simulink model "MATMPC_SIMULINK_SPACEROBOT"  (R2019b)
settings: Solver=ode1  StartTime=0.0  StopTime=10  FixedStep=settings.Ts  RelTol=1e-3
undefined symbols (not defined in the file): indata, opt, settings, x0
libraries: dspindex x3
(part 1 of 2)
settings Model: Creator=chen  LastModifiedBy=ichelikh
settings DataIOCC: ReturnWorkspaceOutputs=off
settings DebuggingCC: ArithmeticOperatorsInVariantConditions=warning
settings SFSimCC: SimUseLocalCustomCode=off  CustomCodeUndefinedFunction=UseInterfaceOnly
settings RTWCC: RTWUseLocalCustomCode=off  CheckMdlBeforeBuild=Error

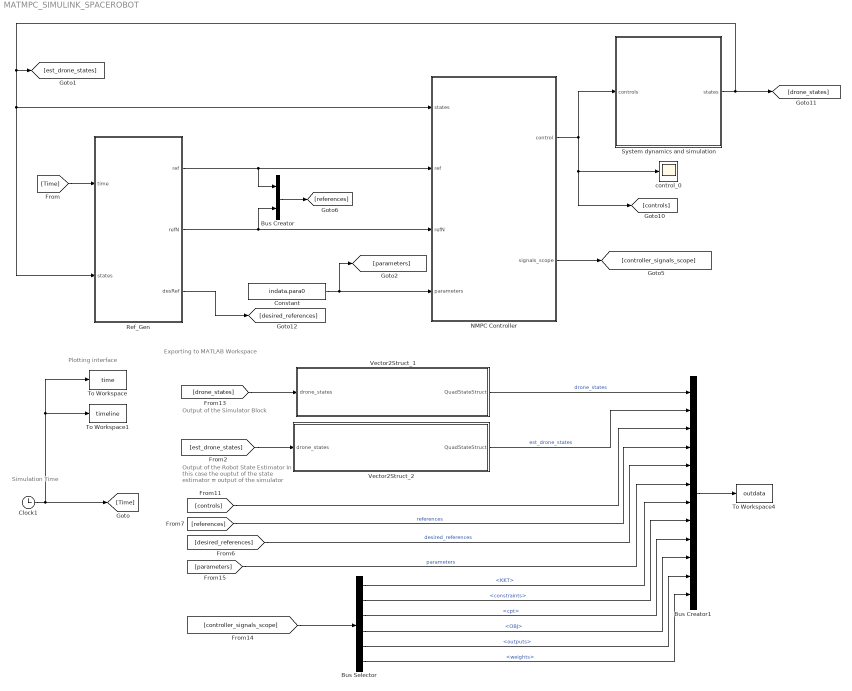
== system MATMPC_SIMULINK_SPACEROBOT ==
  note: Output of the Robot State Estimator
      | In this case the ouptut of the
      | state estimator = output of
      | the simulator
  note: Output of the Simulator Block
  note: Exporting to MATLAB Workspace
  note: Simulation Time
  note: Plotting interface
  Bus Creator : BusCreator  Inputs=2
  Bus Creator1 : BusCreator  Inputs=12
  Bus Selector : BusSelector  OutputSignals=KKT,constraints,cpt,OBJ,outputs,weights
  Clock1 : Clock
  Constant : Constant  Value=indata.para0
  NMPC Controller : Subsystem
  Ref_Gen : Subsystem
  System dynamics and simulation : Subsystem
  To Workspace : ToWorkspace  VariableName=time  SampleTime=-1
      settings: MaxDataPoints=1
  To Workspace1 : ToWorkspace  VariableName=timeline  SampleTime=-1
  To Workspace4 : ToWorkspace  VariableName=outdata  SaveFormat=Timeseries  SampleTime=-1
  Vector2Struct_1 : Subsystem
  Vector2Struct_2 : Subsystem
  control_0 : Scope
  wires:
  NMPC Controller/1(control) -> [controls], control_0/1, System dynamics and simulation/1("controls ")
  Ref_Gen/1(ref) -> Bus Creator/1, NMPC Controller/2("ref ")
  Ref_Gen/2(refN) -> Bus Creator/2, NMPC Controller/3("refN ")
  Constant/1 -> [parameters], NMPC Controller/4(parameters)
  [Time] -> Ref_Gen/1(time)
  Vector2Struct_2/1(QuadStateStruct) -> Bus Creator1/2  "est_drone_states"
  Bus Selector/6 -> Bus Creator1/12  "<weights>"
  Bus Selector/4 -> Bus Creator1/10  "<OBJ>"
  Bus Selector/3 -> Bus Creator1/9  "<cpt>"
  [desired_references] -> Bus Creator1/5  "desired_references"
  [parameters] -> Bus Creator1/6  "parameters"
  [references] -> Bus Creator1/4  "references"
  [controls] -> Bus Creator1/3
  [est_drone_states] -> Vector2Struct_2/1(drone_states)
  Bus Creator1/1 -> To Workspace4/1
  Bus Selector/1 -> Bus Creator1/7  "<KKT>"
  Bus Selector/5 -> Bus Creator1/11  "<outputs>"
  Vector2Struct_1/1(QuadStateStruct) -> Bus Creator1/1  "drone_states"
  Bus Selector/2 -> Bus Creator1/8  "<constraints>"
  [controller_signals_scope] -> Bus Selector/1
  [drone_states] -> Vector2Struct_1/1(drone_states)
  Ref_Gen/3("desRef ") -> [desired_references]
  NMPC Controller/2(signals_scope) -> [controller_signals_scope]
  Bus Creator/1 -> [references]
  System dynamics and simulation/1(states) -> [drone_states], Ref_Gen/2("states "), NMPC Controller/1("states "), [est_drone_states]
  Clock1/1 -> [Time], To Workspace/1, To Workspace1/1

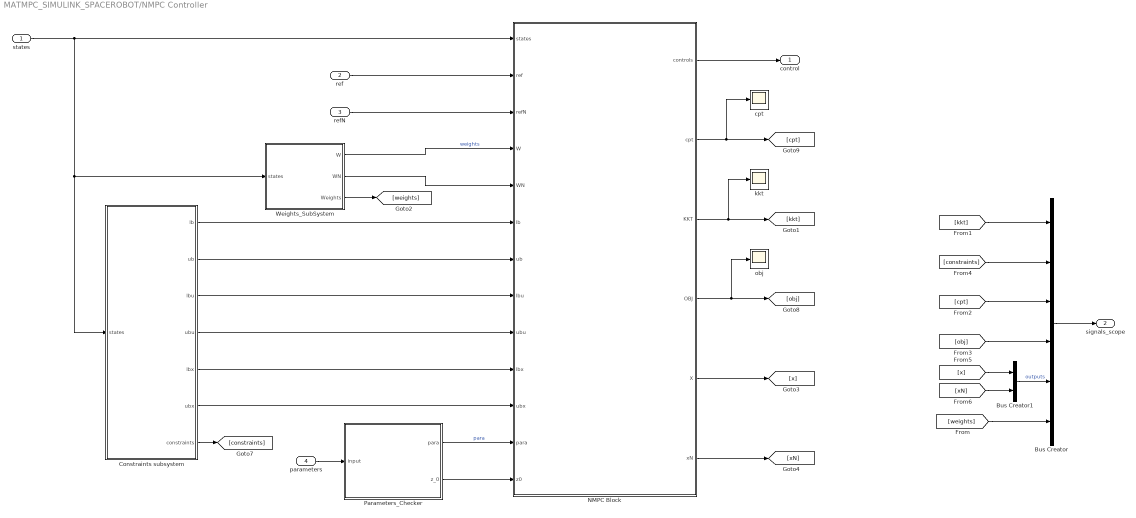
== system MATMPC_SIMULINK_SPACEROBOT/NMPC Controller ==
  "states " : Inport
  "ref " : Inport  Port=2
  "refN " : Inport  Port=3
  parameters : Inport  Port=4
  Bus Creator : BusCreator  Inputs=6
  Bus Creator1 : BusCreator  Inputs=2
  Constraints subsystem : Subsystem
  "NMPC Block " : MATLAB Function  TreatAsAtomicUnit=on  SystemSampleTime=settings.Ts
  Parameters_Checker : MATLAB Function  TreatAsAtomicUnit=on  SystemSampleTime=settings.Ts
  Weights_SubSystem : Subsystem
  cpt : Scope
  kkt : Scope
  obj : Scope
  control : Outport
  signals_scope : Outport  Port=2  VectorParamsAs1DForOutWhenUnconnected=off
  wires:
  "refN "/1 -> "NMPC Block "/3(refN)
  "NMPC Block "/4(OBJ) -> obj/1, [obj]
  "NMPC Block "/3(KKT) -> kkt/1, [kkt]
  "NMPC Block "/2(cpt) -> cpt/1, [cpt]
  "ref "/1 -> "NMPC Block "/2(ref)
  "NMPC Block "/1(controls) -> control/1
  "states "/1 -> Constraints subsystem/1(states), Weights_SubSystem/1(states), "NMPC Block "/1(states)
  Weights_SubSystem/2(WN) -> "NMPC Block "/5(WN)
  Weights_SubSystem/1(W) -> "NMPC Block "/4(W)  "weights"
  Constraints subsystem/1(lb) -> "NMPC Block "/6(lb)
  Constraints subsystem/2(ub) -> "NMPC Block "/7(ub)
  Constraints subsystem/3(lbu) -> "NMPC Block "/8(lbu)
  Constraints subsystem/4(ubu) -> "NMPC Block "/9(ubu)
  Constraints subsystem/5(lbx) -> "NMPC Block "/10(lbx)
  Constraints subsystem/6(ubx) -> "NMPC Block "/11(ubx)
  Parameters_Checker/1(para) -> "NMPC Block "/12(para)  "para"
  parameters/1 -> Parameters_Checker/1(input)
  Parameters_Checker/2(z_0) -> "NMPC Block "/13(z0)
  [x] -> Bus Creator1/1
  [xN] -> Bus Creator1/2
  [kkt] -> Bus Creator/1
  [obj] -> Bus Creator/4
  Bus Creator/1 -> signals_scope/1
  Weights_SubSystem/3(Weights) -> [weights]
  Constraints subsystem/7(constraints) -> [constraints]
  "NMPC Block "/5(X) -> [x]
  "NMPC Block "/6(xN) -> [xN]
  [constraints] -> Bus Creator/2
  [cpt] -> Bus Creator/3
  Bus Creator1/1 -> Bus Creator/5  "outputs"
  [weights] -> Bus Creator/6

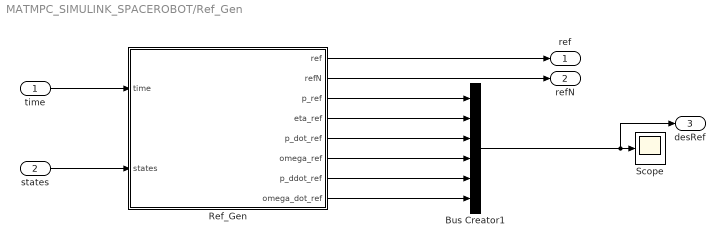
== system MATMPC_SIMULINK_SPACEROBOT/Ref_Gen ==
  time : Inport
  "states " : Inport  Port=2
  Bus Creator1 : BusCreator  Inputs=6
  Ref_Gen : MATLAB Function  TreatAsAtomicUnit=on  SystemSampleTime=settings.Ts
  Scope : Scope
  ref : Outport
  refN : Outport  Port=2
  "desRef " : Outport  Port=3
  wires:
  Ref_Gen/4(eta_ref) -> Bus Creator1/2
  Ref_Gen/3(p_ref) -> Bus Creator1/1
  Ref_Gen/8(omega_dot_ref) -> Bus Creator1/6
  Ref_Gen/2(refN) -> refN/1
  time/1 -> Ref_Gen/1(time)
  Ref_Gen/7(p_ddot_ref) -> Bus Creator1/5
  Ref_Gen/1(ref) -> ref/1
  Ref_Gen/5(p_dot_ref) -> Bus Creator1/3
  Ref_Gen/6(omega_ref) -> Bus Creator1/4
  Bus Creator1/1 -> "desRef "/1, Scope/1
  "states "/1 -> Ref_Gen/2(states)

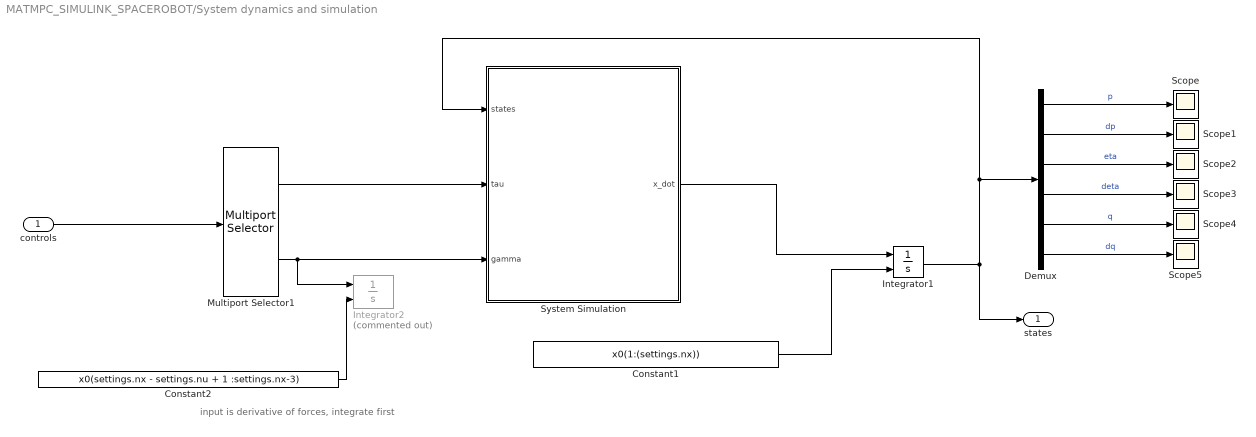
== system MATMPC_SIMULINK_SPACEROBOT/System dynamics and simulation ==
  note: input is derivative of forces, integrate first
  "controls " : Inport
  Constant1 : Constant  Value=x0(1:(settings.nx))
  Constant2 : Constant  Value=x0(settings.nx - settings.nu + 1 :settings.nx-3)
  Demux : Demux  Outputs=6
  Integrator1 : Integrator  InitialConditionSource=external
  Integrator2 : Integrator  Commented=on  InitialConditionSource=external
  Multiport Selector1 : dspindex/Multiport Selector  rowsOrCols=Rows  idxCellArray={settings.nu_lambda + 1 : settings.nu, 1:settings.nu_lambda}  idxErrMode=Clip Index
  Scope{,1..5} (6 alike) : Scope
  System Simulation : MATLAB Function  TreatAsAtomicUnit=on  SystemSampleTime=settings.Ts
  states : Outport
  wires:
  Integrator1/1 -> System Simulation/1(states), Demux/1, states/1
  Constant2/1 -> Integrator2/2
  Demux/1 -> Scope/1  "p"
  Demux/2 -> Scope1/1  "dp"
  Demux/3 -> Scope2/1  "eta"
  Demux/4 -> Scope3/1  "deta"
  Demux/5 -> Scope4/1  "q"
  Demux/6 -> Scope5/1  "dq"
  Constant1/1 -> Integrator1/2
  "controls "/1 -> Multiport Selector1/1
  Multiport Selector1/2 -> Integrator2/1, System Simulation/3(gamma)
  Multiport Selector1/1 -> System Simulation/2(tau)
  System Simulation/1(x_dot) -> Integrator1/1

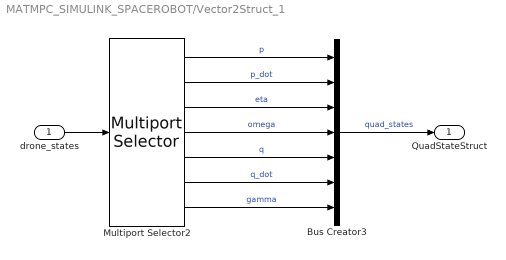
== system MATMPC_SIMULINK_SPACEROBOT/Vector2Struct_1 ==
  drone_states : Inport
  Bus Creator3 : BusCreator  Inputs=7
  Multiport Selector2 : dspindex/Multiport Selector  rowsOrCols=Rows  idxCellArray={ 1:3, 4:6, 7:9, 10:12, 13:15, 16:18, 19:19+settings.nu-1}  idxErrMode=Clip Index
  QuadStateStruct : Outport  VectorParamsAs1DForOutWhenUnconnected=off
  wires:
  Multiport Selector2/2 -> Bus Creator3/2  "p_dot"
  drone_states/1 -> Multiport Selector2/1
  Multiport Selector2/3 -> Bus Creator3/3  "eta"
  Bus Creator3/1 -> QuadStateStruct/1  "quad_states"
  Multiport Selector2/1 -> Bus Creator3/1  "p"
  Multiport Selector2/4 -> Bus Creator3/4  "omega"
  Multiport Selector2/5 -> Bus Creator3/5  "q"
  Multiport Selector2/6 -> Bus Creator3/6  "q_dot"
  Multiport Selector2/7 -> Bus Creator3/7  "gamma"

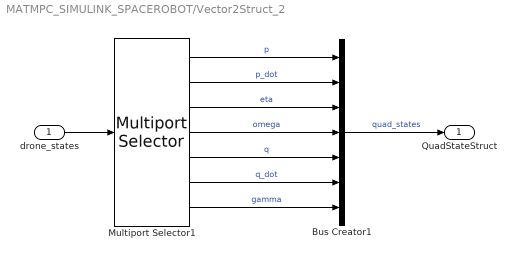
== system MATMPC_SIMULINK_SPACEROBOT/Vector2Struct_2 ==
  drone_states : Inport
  Bus Creator1 : BusCreator  Inputs=7
  Multiport Selector1 : dspindex/Multiport Selector  rowsOrCols=Rows  idxCellArray={ 1:3, 4:6, 7:9, 10:12, 13:15, 16:18, 19:19+settings.nu-1}  idxErrMode=Clip Index
  QuadStateStruct : Outport  VectorParamsAs1DForOutWhenUnconnected=off
  wires:
  Multiport Selector1/6 -> Bus Creator1/6  "q_dot"
  Multiport Selector1/1 -> Bus Creator1/1  "p"
  Multiport Selector1/7 -> Bus Creator1/7  "gamma"
  Multiport Selector1/3 -> Bus Creator1/3  "eta"
  Multiport Selector1/2 -> Bus Creator1/2  "p_dot"
  Multiport Selector1/5 -> Bus Creator1/5  "q"
  Multiport Selector1/4 -> Bus Creator1/4  "omega"
  Bus Creator1/1 -> QuadStateStruct/1  "quad_states"
  drone_states/1 -> Multiport Selector1/1

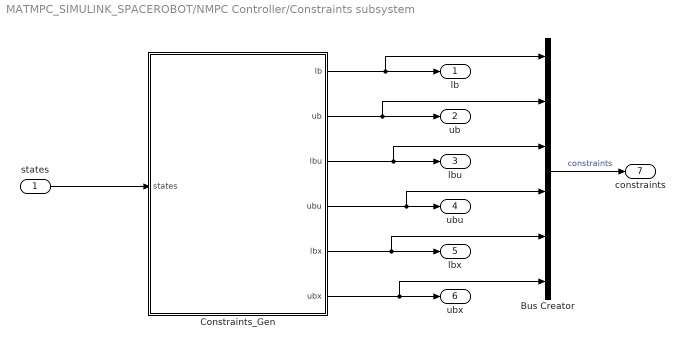
== system MATMPC_SIMULINK_SPACEROBOT/NMPC Controller/Constraints subsystem ==
  states : Inport
  Bus Creator : BusCreator  Inputs=6
  Constraints_Gen : MATLAB Function  TreatAsAtomicUnit=on  SystemSampleTime=settings.Ts
  lb : Outport  VectorParamsAs1DForOutWhenUnconnected=off
  ub : Outport  Port=2  VectorParamsAs1DForOutWhenUnconnected=off
  lbu : Outport  Port=3  VectorParamsAs1DForOutWhenUnconnected=off
  ubu : Outport  Port=4  VectorParamsAs1DForOutWhenUnconnected=off
  lbx : Outport  Port=5  VectorParamsAs1DForOutWhenUnconnected=off
  ubx : Outport  Port=6  VectorParamsAs1DForOutWhenUnconnected=off
  constraints : Outport  Port=7
  wires:
  states/1 -> Constraints_Gen/1(states)
  Constraints_Gen/5(lbx) -> Bus Creator/5, lbx/1
  Constraints_Gen/3(lbu) -> Bus Creator/3, lbu/1
  Constraints_Gen/6(ubx) -> Bus Creator/6, ubx/1
  Constraints_Gen/1(lb) -> Bus Creator/1, lb/1
  Constraints_Gen/2(ub) -> Bus Creator/2, ub/1
  Constraints_Gen/4(ubu) -> Bus Creator/4, ubu/1
  Bus Creator/1 -> constraints/1  "constraints"

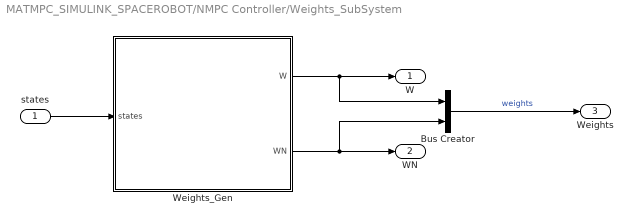
== system MATMPC_SIMULINK_SPACEROBOT/NMPC Controller/Weights_SubSystem ==
  states : Inport
  Bus Creator : BusCreator  Inputs=2
  Weights_Gen : MATLAB Function  TreatAsAtomicUnit=on  SystemSampleTime=settings.Ts
  W : Outport  VectorParamsAs1DForOutWhenUnconnected=off
  WN : Outport  Port=2
  Weights : Outport  Port=3
  wires:
  Weights_Gen/1(W) -> Bus Creator/1, W/1
  states/1 -> Weights_Gen/1(states)
  Weights_Gen/2(WN) -> Bus Creator/2, WN/1
  Bus Creator/1 -> Weights/1  "weights"

== matlab function MATMPC_SIMULINK_SPACEROBOT/System dynamics and simulation/System Simulation ==
  data: x_dot output; states input; tau input size=[settings.nu_m 1]; gamma input size=[settings.nu_lambda 1]; indata parameter
function x_dot  = Dynamic_System(states, tau, gamma,   indata)

%addpath('/home/ichelikh/ms2021-idriss_chelikh/Software/robotics')

%% Dimensions
%nu = 9;  % No. of controls

nu_m = 3; %No. of controls : torques of robot arm actuators
nu_v = 0;       % No. of controls: servo_angle_rates
nu_lambda = 6;      % No. of controls: actuator_force_derivatives
nu = nu_lambda + nu_v+nu_m;  % No. of controls

%% Constraints on state - number and indices


%% Constraints on input - number and indices
nbu = nu;


%% Vectors for system equation

%% Variables definition
% State variables definition
x = states(1);
y = states(2);
z = states(3);
u = states(4);  
v = states(5);
w = states(6);
phi = states(7);
theta = states(8);
psi = states(9);
p = states(10);
q = states(11);
r = states(12);
q1 = states(13);
q2 = states(14);
q3 = states(15);
dq1 = states(16);
dq2 = states(17);
dq3 = states(18);
% f1 = states(19);
% f2 = states(20);
% f3 = states(21);
% f4 = states(22);
% f5 = states(23);
% f6 = states(24);

%% ------------------------------MODELLING--------------------------------
%
% ------------------------------------------------------------------------

% -------------------------------------------------------------------------
% Define the DH parameters
N_DOFS = 3;
dh.theta = zeros(3, 1);
dh.alpha = [pi/2 0 0];

dh.d = [0 0 0];
dh.a = [0 0.3 0.3];
dh.type = ['r' 'r' 'r'];

% -------------------------------------------------------------------------
% Rigid body paramaters: inertia, mass, and center of mass
I1 = diag([0.0005  0.000011 0.0004]);
I2 = diag([0.00035 0.0018   0.0016]);
I3 = diag([0.423   1.414    1.185])*1e-4;
rb.I =  repmat(eye(3), 1, 1, N_DOFS);

rb.I(:,:,1) = I1;
rb.I(:,:,2) = I2;
rb.I(:,:,3) = I3;

rb.m = [0.059 0.256 0.093];
rb.mdrone = 2.122+0.512;
rb.I_drone = diag([0.0115,  0.0114, 0.0194]);

% In standard DH, COM is mesured respect to its end-effector (using local
% frame). When COM is [0 0 0]', it means the COM is located exactly at the
% end-effector. Therefore, COM usually has negative values, which means the
% COM is behind the end-effector

rb.r = [0 0 0; -0.15 0 0; -0.15 0 0]';
rb.rc0 = [0;0;-0.051];
rb.rc1 = [0;0;0];



Gdrone = [ -0.2449    0.2673   -0.2832    0.2496    0.6017   -0.5546
            0.4993   -0.4947   -0.4691    0.4971    0.0212   -0.0038
            0.7157    0.6958    0.6572    0.6714    0.7051    0.7304
           -0.0031    0.1762    0.1769   -0.0046   -0.1827   -0.1746
           -0.2100   -0.0996    0.0945    0.2112    0.1111   -0.1077
            0.1976   -0.1857    0.1864   -0.1945    0.1894   -0.1923 ];

epsilon = [states(1:3); states(7:9); states(13:15)]; % eps = [xb, phib, q]

depsilon = [states(4:6); states(10:12); states(16:18)]; % deps = [vb, dphib, dq]

phib = epsilon(4:6)';
wRb = att2RotMat('xyz', phib);

Gdrone = [wRb*Gdrone(1:3,:);
          Gdrone(4:6,:)];

Gforces = Gdrone*gamma;
Big_Eye = eye(9);

G_C_Mat = invdyn(dh, rb, epsilon, depsilon, zeros(9,1),[0; 0; -9.8]);

M = zeros(9,9);

for i = 1:nu
    M(:,i) = invdyn(dh, rb, epsilon, zeros(9,1), Big_Eye(i,:)', [0; 0; 0]);
end 

real_u = [Gforces;tau];

epsilon_ddot = M\(real_u-G_C_Mat);
%

T_plate = [1 cos(phi)*tan(theta)  sin(phi)*tan(theta);
           0 cos(phi)            -sin(phi);
           0 sin(phi)/cos(theta)  cos(phi)/cos(theta)];     
       
v_all   = [u;v;w];
acc_all = epsilon_ddot(1:3); 
att_dot = T_plate*[p;q;r];
domega  = epsilon_ddot(4:6);
dq      = [dq1; dq2; dq3];
ddq     = epsilon_ddot(7:9); 


x_dot   = [
        v_all;
        acc_all;
        att_dot;
        domega;
        dq;
        ddq;
        ];
    
end
%% -----------------FUNCTIONS USED FOR MODEL COMPUTATION-------------------

% -------------------------------------------------------------------------
function Qtot = invdyn(dh, rb, epsilon, depsilon, ddepsilon,  grav)
% Inverse dynamic with recursive Newton-Euler following De luca slides

if nargin < 6
    grav = [0;0;0];
end

z0 = [0; 0; 1];


bwb    = depsilon(4:6);  %omega of base com in base frame
wdotb = ddepsilon(4:6); %omega dot of base com in base frame
a0b   = ddepsilon(1:3); %p ddot of base com in world frame

q     = epsilon(7:end); 
qdot  = depsilon(7:end);
qddot = ddepsilon(7:end);


% init all to sx zeros
w     = zeros(3,3);
wdot  = zeros(3,3);
vdot  = zeros(3,3);

n     = zeros(3,3);
f     = zeros(3,3);

z     = zeros(3,3);

Q     = zeros(3,1);
N_DOFS = length(q);
%Rb = eye(3);

R0b= [0 1 0;
      0 0 1;
      1 0 0];

%init with respect of world frame

phib = epsilon(4:6)'; %yaw-pitch-roll Euler angles (moving)
wRb = att2RotMat('xyz', phib);
p0b = [0; 0; -0.05];  % offset between link 0 and com in BASE frame

% omega and omega dot of base in world frame
wwb= wRb*bwb;
wdotwb = wRb*wdotb;
%acc resultant of 1st link frame 0 with respect of worldframe
w_a0 = a0b + cross(wdotwb , (wRb*p0b)) + cross(wwb, cross(wwb, wRb*p0b)) - grav; % premulitply with rotations
% you need to rotate in frame 0 the gravity (which is expressed in world frame) 
a0 = R0b*wRb'*w_a0;
w0 = R0b*bwb; 
wdot0 = R0b*wdotb;
    % ---------------------------------------------------------------------
    % Forward recursion 
    for i = 1 : N_DOFS
        T = calc_transformation(i-1, i, dh, q);
        R = T(1:3, 1:3);
        %R0 = R0*R;
        p = [dh.a(i); dh.d(i)*sin(dh.alpha(i)); dh.d(i)*cos(dh.alpha(i))];
        %z = R*z0;
        if i > 1
            
            z(:,i)    =  z0;%(:,i-1);
            w(:,i)    =  R'*(w(:,i-1) + z0.*qdot(i));
            
            wdot(:,i) =  R'*(wdot(:,i-1) +  z0.*qddot(i) + ...
                         cross(w(:,i-1), z0.*qdot(i)));
                    
            vdot(i,:) =  R'*vdot(:,i-1) + cross(wdot(:,i), p) + ...
                         cross(w(:,i-1), cross(w(:,i),p));
        else
            z(:,i)    =  z0;
            w(:,i)    =  R'*(w0 + z0.*qdot(i));
            
            wdot(:,i) =  R'*(wdot0 + z0.*qddot(i) + ...
                         cross(w0, z0.*qdot(i)));
            
            vdot(:,i) =  R'*(a0) + cross(wdot(:,i), p) + ...
                         cross(w(:,i), cross(w(:,i),p));
        end
    end
    
    z0 = [0; 0; 1];
    
    % Dynamic simulation
    % Backward recursion
    for i = N_DOFS:-1:1
        p = [dh.a(i); dh.d(i)*sin(dh.alpha(i)); dh.d(i)*cos(dh.alpha(i))];
        
        vcdot = vdot(:,i) + cross(wdot(:,i),rb.r(:,i)) + ...
                cross(w(:,i),cross(w(:,i),rb.r(:,i)));
        
        F = rb.m(i)*vcdot;
        N = rb.I(:,:,i)*wdot(:,i)+cross(w(:,i),rb.I(:,:,i)*w(:,1));
        
        if i < N_DOFS
            T = calc_transformation(i, i+1, dh, q);
            R = T(1:3, 1:3);
            
            n(:,i) = R*(n(:,i+1) + cross(R'*p, f(:,i+1))) + ...
                     cross(rb.r(:,i)+p,F) + N;
                 
            f(:,i) = R*f(:,i+1) + F;
        else
            n(:,i) = cross(rb.r(:,i)+p,F) + N;
            f(:,i) = F;
        end
        
        T = calc_transformation(i-1, i, dh, q);
        R = T(1:3, 1:3);
      % z0 = [0;0;1];
        if dh.type(i) == 't'
            Q(i) = f(:,i)'*R'*z0;
        elseif dh.type(i) == 'r'
            Q(i) = n(:,i)'*R'*z0;
        end
    end

    wrenchB = wrench_base(f(:,1), n(:,1), R0b, p0b, w0, rb.mdrone, rb.I_drone, ddepsilon, grav);
    
    Qtot = [wrenchB;Q];
    
end

function [wrench] = wrench_base(f0, n0, Rb0, p0b, bwb, m, J, ddepsilon, grav)

%   RotWM = [Rw0,      zeros(3,3);
%            zeros(3,3), eye(3)];
  RotWM = eye(6);

  Mass  = [ m*eye(3),  zeros(3,3); 
            zeros(3,3),        J];
  
  RotM0 = [[eye(3)         , zeros(3,3)];
           [skewMat(p0b), Rb0       ]];
  
  f0 = Rb0'*f0;
  n0 = Rb0'*n0;
  
  wrench0 = [f0; n0];
  
  gyro = -cross(bwb, J*bwb);
  
  Grav_and_Gyro = [m*grav ; gyro];
  
  acc = ddepsilon(1:6);

  wrench =  RotWM*(Mass*acc - Grav_and_Gyro - RotM0*wrench0);
end
% -------------------------------------------------------------------------
function  T = calc_transformation(from, to, dh, qc)
% Transformation from one joint to another joint
% 0<=from<N_DOFS
% 0<to<=N_DOFS

T = eye(4);
N_DOFS = length(qc);

% Sanity check
if (from >= N_DOFS) || (from < 0) || (to <= 0) || (to >  N_DOFS)
    return;
end

for i = from+1 : to
    if     dh.type(i) == 'r'
           dh.theta(i) = qc(i);
    elseif dh.type(i) == 'p'
           dh.d(i) = qc(i);
    end

    ct = cos(dh.theta(i));
    st = sin(dh.theta(i));
    ca = cos(dh.alpha(i));
    sa = sin(dh.alpha(i));
    
    T = T * [ ct    -st*ca   st*sa     dh.a(i)*ct ; ...
              st    ct*ca    -ct*sa    dh.a(i)*st ; ...
              0     sa       ca        dh.d(i)    ; ...
              0     0        0         1          ];
          
end
end





%% motion dynamics parameters definition
% J = indata.model.J;
% m = indata.model.m;
% Gdrone = indata.model.G;
% % Gravity [m/s^2]
% % p     = [x; y; z];  Not needed: kept for consistency
% % p_dot = [u, v, w];  Not needed: kept for consistency
% % eta   = [phi; theta; psi];
% % omega = eta_dot = [p; q; r];
% % gamma = f = [f1; f2; f3; f4; f5; f6];
% 
% %% Extract variables
% %robot1 = indata.robot;
% % ... from eta vector: needed to compute matrices R and T
% x = pos(1);
% y = pos(2);
% z = pos(3);
% 
% u = p_dot(1);
% v = p_dot(2);
% w = p_dot(3);
% 
% phi = eta(1);
% theta = eta(2);
% psi = eta(3);
% 
% p = omega(1);
% q = omega(2);
% r = omega(3);
% 
% q1 = q_an(1);
% q2 = q_an(2);
% q3 = q_an(3);
% 
% dq1 = dq(1);
% dq2 = dq(2);
% dq3 = dq(3);
% % 
% % B = compute_inertia(phi, theta, psi, q1,q2,q3);
% % 
% G = compute_gravity_vect(theta, phi, q1,q2,q3);
% % 
% % 
% 
% 
% % % Initialize 
% n = 3;             
% % Only n firsts elements of the
% % following vectors might be
% % used: thus define next vectors accordingly!
%  joint_types = ['r' 'r' 'r']; 
% % type of joint j. Valid values are: 'r':rotational, 'p':prismatic
% 
% %% ~~~~~~~~~~~~~~~~~~~~~~~~ DH PARAMETERS ~~~~~~~~~~~~~~~~~~~~~~~~ 
% a = [0 0.3 0.3]; d = [0 0 0]; alpha = [pi/2 0 0]; angles = [q1 q2 q3];
% 
% % Values of the DH parameters when the robot1 is in its home (rest) pose
% theta1 = [pi 0 0];
% 
% % Derivatives of the DH parameters 
% dtheta = [dq1 dq2 dq3];
% 
% %% ~~~~~~~~~~~~~~~~~~~~~~~~ KINEMATICS ~~~~~~~~~~~~~~~~~~~~~~~~ % pl:
% % position of the c.o.m of Link i wrt Link Frame i (knwon at priori, depend
% % upon robot1's mechanical design) 
% values_pl = [[0; 0; 0] [-0.3/2; 0; 0] [-0.3/2; 0; 0]];
% 
% % Position and orientation of Frame B wrt World Frame W 
% pwb = [x; y; z];
% phib = [psi; theta; phi]; %yaw-pitch-roll Euler angles (moving) 
% Rwb = att2RotMat('zyx', phib);
% 
% % Linear and Angular velocities of Body wrt World Frame W 
% dpwb = [u; v;w]; dphib = [p; q; r];
% 
% % Position and orientation of Manipulator's Frame 0 wrt Body Frame B pb0 = [xb0 yb0 zb0]'; 
%  pb0 = [0 0 0.1]'; 
%  
% Rb0 = att2RotMat('zyx', [-pi/6 -pi/2 -pi/2]);
% 
% 
% Twb = [ cos(theta)*cos(psi)  -sin(psi)  0;
%         cos(theta)*sin(psi)   cos(psi)  0;
%              -sin(theta)        0       1 ];
%          
% Qwb = (Rwb') * Twb;
% 
% % Generalised joint vector 
% epsilon = [ pwb; phib; angles' ];
%                 
% depsilon = [ dpwb; dphib; dtheta' ];
% 
% %% Compute Homogenous Transformation Matrices From Link Frame i-1 to LinkFrame i 
% A = HTML2L(a, d, alpha, angles);
% % A contains the homogeneous transformation matrices from link i-1 to link i. 
% % In the case of the=3dof arm, i is in {1, 2, 3}, where i = 3 is the 
% % end-effector "link", and Frame 0 denotes the "base" of the manipulator.
%                  
% %% Compute Links quantities disp(''); disp('Preliminary kinematic quantities:');
% 
% m = 2.771; % weight with the battery indata.m = m;
% 
% g = 9.81;
% 
% % Inertia [kg*m^2] 
% Ix = 0.083; Iy = 0.081; Iz = 0.16;
% 
% Hb = diag([Ix, Iy, Iz]); % inertial matrix of drone 
% mb = indata.m; %kg mass of drone
% 
% 
% H1 = diag([0.00005, 0.000011, 0.00004]);
% H2 = diag([0.00035, 0.002   , 0.0016]);
% H3 = diag([4.23e-5, 1.41e-4 , 1.19e-4]);
% 
% H_arm = zeros(3,3,n);%inertia matrixes of arms bodies
% 
% H_arm(:,:,1)= H1;
% H_arm(:,:,2)= H2;
% H_arm(:,:,3)= H3;
% 
% 
% m_arm = [0.06 0.256 0.093];
% 
% R    = zeros(3,3,n); posi = zeros(3,1,n);
% 
% pl  = zeros(3,1,n);
% 
% p0  = zeros(3,1,n); R0  = zeros(3,3,n);
% 
% pb  = zeros(3,1,n); Rb  = zeros(3,3,n);
% 
% z0  = zeros(3,1,n); zb  = zeros(3,1,n);
% zb0  = zeros(3,1);
% pbl = zeros(3,1,n);
% 
% for i = 0 : n
%   
%   if i == 0 % ------------ { base }
% 
%     H = Hb; m = mb;
%     
%     % Z-axis coordinates of Base Frame 0 wrt Body Frame B 
%     zb0 = Rb0 * [0; 0; 1];
%   
%   else % ------------ { link }
%     %fprintf('* for link %d\n', i); % Inertia (expressed wrt Link Frame i)and mass of Link i
%     H = H_arm(:,:,i);
%     m = m_arm(i);
% 
%     % Get Homogeneous Transformation Matrix from Link Frame i-1 to Link 
%     %Frame i 
%     A_i = A(1+(i-1)*4:4+(i-1)*4,:); 
%     % Get position andorientation of Link Frame i wrt Link Frame i-1 (DH % Parameters)
%     R(:,:,i) = A_i(1:3, 1:3); 
%     posi(:,:,i) = A_i(1:3, 4);
%     
%     % Position of the c.o.m of Link i wrt Link Frame i
%       pl(:,:,i) = values_pl(:,i);
%     
%     % Position and orientation of Link Frame i wrt Link Base Frame 0 
%     if i == 1 % ------------ { first link }
%       p0(:,:,i) = posi(:,:,i); 
%       R0(:,:,i) = R(:,:,i);
% 
%     else % ------------ { i-th link }
%       p0(:,:,i) = p0(:,:,i-1) + R0(:,:,i-1) * posi(:,:,i); 
%       R0(:,:,i) = R0(:,:,i-1) * R(:,:,i);
%       
%     end
%     
%     % Position and orientation of Link Frame i wrt Body Frame B 
%     pb(:,:,i) = pb0 + Rb0 * p0(:,:,i);
%   
%     Rb(:,:,i) = Rb0 * R0(:,:,i);
% 
%     % Z-axis coordinates of Link Frame i wrt Base Frame 0 
%     %   [0; 0; 1] = zi 
%     %   zi: z-axis coordinates of Link Frame i wrt Link Frame i
%     z0(:,:,i) = R0(:,:,i) * [0; 0; 1];
%     
%     % Z-axis coordinates of Link Frame i wrt Body Frame B 
%     zb(:,:,i) = Rb0 * z0(:,:,i);
% 
%     % Position of the c.o.m of Link i wrt Body Frame B 
%     pbl(:,:,i) = pb(:,:,i) + Rb(:,:,i) * pl(:,:,i);
%   end
%          
% end
% 
% %% Kinematics 
% 
% disp(''); 
% disp('Kinematics:')
% 
% J   = zeros(6,n,n); 
% S   = zeros(3,3,n); 
% Hbl = zeros(3,3,n);
% 
% for i = 1:n % cycle over links
%   %fprintf('* Jacobian of link %d\n', i);
%   
%   %Ji = sym('j%d%d', [6 n], 'real');
%   Ji   = zeros(6,n);
%   for j = 1:n % ------------ { cycle over joints (columns of each Linki's Jacobian) }
% 
%     if j <= i % ------------ { Effects of Links before i or i itself }
% 
%       if j == 1 % ------------ { first joint }
%         switch lower(joint_types(j))
%           case 'p'
%             Ji(:,j) = [ zb0;
%                         zeros(3,1)
%                       ];
%           case 'r'
%             Ji(:,j) = [ cross((zb0), (pbl(:,:,j) - pb0)); %ijacobian computation using pluckerian coords
%                         zb0
%                       ];
%           otherwise
%             %fprintf('Joint %d\n', j); error('Invalid joint type');
%         end
% 
%       else % ------------ { j-th joint }
%         switch lower(joint_types(j))
%           case 'p'
%             Ji(:,j) = [ zb(:,:,j-1);
%                         zeros(3,1)
%                       ];
%           case 'r'
%             Ji(:,j) = [ cross(zb(:,:,j-1), (pbl(:,:,j-1)- pb(:,:,j-1)));
%                               zb(:,:,j-1)
%                         ];
%           otherwise
%             %fprintf('Joint %d\n', j); error('Invalid joint type');
%         end
%       end
% 
%     else % ------------ { Effects of Links after i }
%       Ji(:,j) = zeros(6, 1);
%     end
%   end
%   
%   Si = skewMat(Rwb * pbl(:,:,i)); 
%   
%   Hbli = Rb(:,:,i) * H_arm(:,:,i) * (Rb(:,:,i)');
%   
%   J(:,:,i)    = Ji; 
%   S(:,:,i)    = Si; 
%   Hbl(:,:,i)  = Hbli;
% end
% 
% % Dynamics disp(''); disp('Dynamics:')
% 
% e3 = [0; 0; 1];
% 
% nepsilon = length(epsilon);
% 
% % Get variables related to the Base 
% mb    = m; 
% pb    = pwb; 
% Rb    = Rwb; 
% Tb    = Twb; 
% Qm    = Qwb;
% 
% % Initialize submatrices of Generalised Inertia Matrix B 
% 
% B11 = mb;
% 
% B22 = (Qm') * Hb * Qm;
% 
% B33 = zeros(3,3);
% 
% B12 = zeros(3,3);
% 
% B13 = zeros(3,3);
% 
% B23 = zeros(3,3);
% 
% % Initialize Potential Energy U 
% % U = mb * g * (e3') * pb;
% 
% 
% disp('* Generalised Inertia Matrix B')
% 
% for i = 1:n
%   
%   %fprintf('** Link %d\n', i);
%   
%   % Get variables related to Link i 
%     Jpi   = J(1:3,:,i); 
%     Joi   = J(4:6,:,i); 
%     mi    = m_arm(i); 
%     Si    = S(:,:,i); 
%     Hbli  = Hbl(:,:,i); 
%     pbli  = pbl(:,:,i);
%   
%   B11 = B11 + mi;
%   
%   B22 = B22 ...
%             + mi * (Tb)' * (Si') * Si * Tb + (Qm') * Hbli * Qm;
%   
%   B33 = B33 ...
%             + mi * (Jpi') * Jpi ... 
%             + (Joi') * Hbli * Joi;
%         
%   B12 = B12 ...
%             - mi * (Si) * Tb;
%         
%   B13 = B13 ...
%             + mi * Rb * Jpi;
%   
%   B23 = B23 ...
%             + (Qm') * Hbli * Joi ... 
%             - mi * (Tb') * (Si') * Rb * Jpi;
%           
% %   U = U ...
% %         + mi * g * (e3') * (pb + Rb * pbli);
%           
% end
% 
% % Finalize submatrices 
% B11 = B11 * eye(3);
% 
% 
% % Exploit symmetry of Generalised Inertia Matrix 
% B21 = B12'; B31 = B13';
% B32 = B23';
% 
% % Compose Generalised Inertia Matrix B 
% B = [ B11 B12 B13;
%       B21 B22 B23;
%       B31 B32 B33 ];
% 
% % disp('* Gravitational Vector G') 
% % % G = jacobian(U, epsilon);
% 
% %% compute C matrix Coriolis C = SX.sym('C', nepsilon,nepsilon); for i =
% % 1:nepsilon
% %   
% %   epsiloni = epsilon(i);
% %   
% %   % Fill all columns at row i of Coriolis Matrix C % jacobian(B,epsiloni)
% %   Bk = []; for k =1:nepsilon
% %     Bk = [Bk jacobian(B(:, k),epsiloni)];
% %     
% %   end
% %     Ctemp = 0.5 * (jacobian(B(:,i),epsilon) + jacobian(B(:,i),epsilon).'
% %     - Bk); Ctemp = depsilon.' * Ctemp * depsilon; C(:,i) = Ctemp; % here
% %     you get C*epsilon, which is different from C !!
% % end 
% % allocation matrix of drone base
% 
% Gdrone = [-0.0139,  0.2777, -0.2991, -0.0109,  0.2729, -0.2964;
%            0.3343, -0.1620, -0.1585,  0.3330, -0.1601, -0.1595; 
%            0.9486,  0.9360,  0.9494,  0.9391,  0.9514,  0.9389; 
%            0.0056,  0.3021,  0.3042,  0.0044, -0.2930, -0.2942;
%           -0.3525, -0.1784,  0.1640,  0.3383,  0.1633, -0.1782;
%            0.1247, -0.1661,  0.1234, -0.1681,  0.1227, -0.1668];
% 
% 
% G1 = Gdrone(1:3, :); G2 = Gdrone(4:6, :);
% 
% r11 = cos(theta) * cos(psi); 
% r21 = cos(theta) * sin(psi); 
% r31 = -sin(theta); 
% r12 = sin(phi) * sin(theta) * cos(psi) - cos(phi) * sin(psi); 
% r22 = sin(phi) * sin(theta) * sin(psi) + cos(phi) * cos(psi);
% r32 = sin(phi) * cos(theta); 
% r13 = cos(phi) * sin(theta) * cos(psi) +sin(phi) * sin(psi); 
% r23 = cos(phi) * sin(theta) * sin(psi) - sin(phi) *cos(psi); 
% r33 = cos(phi) * cos(theta);
% 
% R = [[r11 r21 r31].', [r12 r22 r32].', [r13 r23 r33].'];
% 
% G1 = R * G1;
% 
% G_drone = [G1;
%            G2];
% Q_nc = [G_drone,zeros(6, 3) ;
%         zeros(3, 6), eye(3)];
% 
% %diag(A_drone, eye(nu_m));
% %% EoM inversion 
% % 
% 
% controls = [gamma ; tau];
% % neglect C*depsilon 
% 
% ddeps = B\(Q_nc*controls -  G');
% 
% v_all   = [u;v;w];
% acc_all = ddeps(1:3); 
% att     = [p;q;r];
% domega  = ddeps(4:6);
% dq      = [dq1; dq2; dq3];
% ddq     = ddeps(7:9); 
% 
% t11 = 1; t12 = 0;         t13 = -sin(theta);
% t21 = 0; t22 = cos(phi);  t23 = sin(phi)*cos(theta);
% t31 = 0; t32 = -sin(phi); t33 = cos(phi)*cos(theta);
% 
% T = [t11 t12 t13; t21 t22 t23; t31 t32 t33];
% 
% %% Return output
% % p_dot = p_dot; % unnecessary 
% p_ddot = acc_all;
% eta_dot = T \ att;
% omega_dot = domega;

%return

== matlab function MATMPC_SIMULINK_SPACEROBOT/NMPC Controller/NMPC Block  ==
  settings: updateMethod=DISCRETE
  data: states input size=nx; opt parameter; ref input size=[ny N]; refN input size=nyN; controls output size=[nu 1]; cpt output size=1; KKT output; OBJ output; W input; WN input; lb input; ub input; lbu input; ubu input; lbx input; ubx input; settings parameter; para input; z0 input; X output; xN output
function [controls, cpt, KKT, OBJ,X, xN] = NMPC_BLOCK(states, opt, ref, refN, W, WN, lb, ub, lbu, ubu, lbx, ubx, settings, para, z0)

%% everything should has a fixed size
coder.extrinsic('mpc_nmpcsolver_simulink');  
coder.extrinsic('InitData');  
coder.extrinsic('InitMemory');  
coder.extrinsic('evalin');
coder.extrinsic('assignin');

%%

persistent x u z lambda mu mu_x mu_u;
persistent input mem;

if isempty(input)  
    
    nx = settings.nx;        % No. of differential states
    nu = settings.nu;        % No. of controls
    nz = settings.nz;        % No. of algebraic states
    ny = settings.ny;        % No. of outputs (references)    
    nyN= settings.nyN;       % No. of outputs at terminal stage 
    np = settings.np;        % No. of parameters (on-line data)
    nc = settings.nc;        % No. of constraints
    ncN = settings.ncN;      % No. of constraints at terminal stage
    nbu = settings.nbu;      % No. of control bounds
    nbx = settings.nbx;      % No. of state bounds
    nbu_idx = settings.nbu_idx; % Index of control bounds
    nbx_idx = settings.nbx_idx; % Index of state bounds
    N = settings.N;
    N2 = settings.N2;
    r = settings.r;
        
    input.x0=states;
    
    x=repmat(states,1,N+1);
    input.x=x;
    
    u=zeros(nu,N);
    input.u=u;
    
    z=repmat(z0,1,N);
    input.z=z;
    
    lambda = zeros(nx,N+1);
    input.lambda= lambda;
    
    if N*nc+ncN > 0
        mu = zeros(N*nc+ncN,1);
    else
        mu = 0;
    end
    input.mu= mu;
    
    mu_u = zeros(N*nu,1);
    input.mu_u= mu_u;
    
    if N*nbx > 0
        mu_x = zeros(N*nbx,1);
    else
        mu_x = 0;
    end
    input.mu_x = mu_x;
    
    input.W=W;
    input.WN=WN;
    input.od = para;
    
    input.lb = lb;
    input.ub = ub;
    input.lbx = lbx;
    input.ubx = ubx;
    input.lbu = lbu;
    input.ubu = ubu;
      
    input.y = ref;
    input.yN = refN;
    
    mem = InitMemory(settings, opt, input);
        
else
    %lines added for custom purpose (IDRISS)
    input.W=W;
    input.WN=WN;
    input.od = para;
    
    input.lb = lb;
    input.ub = ub;
    input.lbx = lbx;
    input.ubx = ubx;
    input.lbu = lbu;
    input.ubu = ubu;
      
    input.y = ref;
    input.yN = refN;
    %END OF CUSTOM
    
    input.x=x; 
    input.u=u;
    input.z=z;
    input.lambda=lambda;   
    input.mu=mu;
    input.mu_x=mu_x;
    input.mu_u=mu_u;
    
    input.x0 = states;
    
end

%%
cpt = 0;
KKT = 0;
OBJ = 0;

% input.x0 = states;
[input,mem,cpt,KKT,OBJ] = mpc_nmpcsolver_simulink(input, settings, mem, opt);
controls = input.u(:,1);

%% Compute cost function terms
if opt.enable_outputVars
  X = input.x(:, 1:end-1);
  xN = input.x(:, end);       
else
  X = zeros(input.x, N);
  xN = zeros(input.x, 1);
end

%% shifting
switch opt.shifting
    case 'yes'
        x=[input.x(:,2:end),input.x(:,end)];  
        u=[input.u(:,2:end),input.u(:,end)]; 
        z=[input.z(:,2:end),input.z(:,end)]; 
        lambda=[input.lambda(:,2:end),input.lambda(:,end)];
        if (settings.N*settings.nc+settings.ncN) >0
            mu(1:end-settings.ncN+1)=input.mu(settings.nc+1:settings.N*settings.nc+settings.ncN,1);
            mu(settings.N*settings.nc+1:end)=input.mu(settings.N*settings.nc+settings.ncN-settings.nc+1:settings.N*settings.nc+settings.ncN,1);
        else
            mu=0;
        end
        mu_x=[input.mu_x(2:end,1);input.mu_x(end,1)];
        mu_u=[input.mu_u(2:end,1);input.mu_u(end,1)];
   case 'no'
        x=input.x;
        u=input.u;
        z=input.z;
        lambda=input.lambda;
        mu=input.mu;
        mu_x=input.mu_x;
        mu_u=input.mu_u;
end

return

== matlab function MATMPC_SIMULINK_SPACEROBOT/Ref_Gen/Ref_Gen ==
  settings: updateMethod=DISCRETE  sampleTime=settings.Ts
  data: ref output; settings parameter; refN output; time input; states input size=settings.nx; p_ref output; eta_ref output; p_dot_ref output; omega_ref output; p_ddot_ref output; omega_dot_ref output; indata parameter
function [ref, refN, p_ref, eta_ref, p_dot_ref, omega_ref, p_ddot_ref, omega_dot_ref] = Reference_Gen(settings, time, states, indata)

persistent j motion t_start desired_WP dtau dtq W_p_B WPs desired_q qtraj qref ;
            
%% Import variables
% ... from struct "settings"
N = settings.N;
ny = settings.ny;
nyN = settings.nyN;
nu_v = settings.nu_v;
nu_lambda = settings.nu_lambda;
Ts_st = settings.Ts_st;

% ... from vector "data"
x0 = indata.x0;

%% Initialize vectors

curr_pos = zeros(3, 1);
ref = zeros(ny, N);
refN = zeros(nyN, 1);

REF = zeros(ny, (N + 1));

p_ref = zeros(3, 1); 
eta_ref = zeros(3, 1); 
p_dot_ref = zeros(3, 1); 
omega_ref = zeros(3, 1); 
p_ddot_ref = zeros(3, 1); 
omega_dot_ref = zeros(3, 1);

%% Take current state
curr_pos(1) = states(1); % At the beginning states is equal to x0 (see Initialization_Simulink.m)
curr_pos(2) = states(2);
curr_pos(3) = states(3); 

%% Initialize default values for reference trajectory
% Some may be overwritten in next section

% Default values for desired position
x = 0; 
y = 0; 
z = 0;
% Default values for desired linear velocity
x_dot = 0; 
y_dot = 0; 
z_dot = 0;
% Default values for desired attitude
roll = 0; 
pitch = 0;             
yaw = 0; 
% Default values for desired angular velocity
omega_x = 0; 
omega_y = 0; 
omega_z = 0;
% Default values for desired angle pos
q1r = pi; 
q2r = 0; 
q3r = 0;
%[0.2; 0.3; 0.1]
% Default values for desired angle speed
dq1r = 0; 
dq2r = 0; 
dq3r = 0;

x_ddot = 0; 
y_ddot = 0; 
z_ddot = 0;

domega_x = 0; 
domega_y = 0; 
domega_z = 0;

ddq1r = 0; 
ddq2r = 0; 
ddq3r = 0;

  % insert IK algorithm here 

%% Generate reference trajectory
for i = 1: N+1 
  % ........................ Sequence of waypoints ......................
  p_t0 = indata.x0(1:3); % starting position --- p(t=t0)
  h_safe = 0; % safety-height offset
  av_speeds = indata.wps.vel; % import speeds steps
  n_wps = indata.wps.num; % import number of waypoints
  if isempty(desired_WP) && isempty(desired_q)
      j = 1; 
      WPs = indata.wps.pos; % load sequence of waypoints
      qtraj = indata.wps.q;
      desired_q = qtraj(:,j);
      desired_WP = WPs(:,j); % set as desired waypoint the current one
      % initialize body position in World frame (where drone 
      % should be at current time t)
      
      W_p_B = p_t0 + [0; 0; h_safe]; 
      qref  = indata.x0(13:15);
      t_start = indata.wps.t_start; % import time instant in which motion should start
      dtau = 1;
      dtq  = 1;
      motion = 0;
  end
  if (time > t_start) && ~motion && j < n_wps
      desired_WP = WPs(:, j+1); % set as desired waypoint the next one
      desired_q = qtraj(:,j+1);
      distances = sqrt((desired_WP - WPs(:,j)).^2); % compute distance to next waypoint
      qdist     = sqrt((desired_q  - qtraj(:,j)).^2);
      % compute time needed to reach next waypoint using 
      % corresponding constant speed step
      dtau = norm(distances)/ 4.5 / av_speeds(j); 
      dtq  = norm(qdist)/4.5;
      if dtau > 0.001 || dtq > 0.001% if next waypoint if far enough
          motion = 1; % trigger motion
      end
  end

  if motion % if motion has been triggered
      t = (time - t_start) / dtau;
      % compute position where drone should be at current time t,
      % through a 2nd-order system response to motion step
      W_p_B = WPs(:,j) + (desired_WP - WPs(:,j)) .* (1 - exp(-t) - t*exp(-t)); 
      qref  = qtraj(:,j) + (desired_q  - qtraj(:,j)).* (1 - exp(-t) - t*exp(-t)); 
      if norm(W_p_B - desired_WP) < 0.01 % if next waypoint has been reached
          disp('drone waypoint reached');
          disp(j+1);
          j = j+1; % point to next waypoint
          motion = 0; % reset motion trigger
          t_start = time + indata.wps.t_rest; % wait rest time before start next motion step
      end
  end
  % set as desired coordinates the position where drone should be
  % at current time t
  x = W_p_B(1); 
  y = W_p_B(2);
  z = W_p_B(3);
  
  q1r = qref(1); 
  q2r = qref(2); 
  q3r = qref(3);

  % set desired yaw
  yaw = x0(9);

% Return desired reference trajectory of first shooting point for
% plotting purposes
if i == 1
    p_ref = [x y z]';
    p_dot_ref = [x_dot y_dot z_dot]';
%     p_ddot_ref = [x_ddot y_ddot z_ddot]';

    eta_ref = [roll pitch yaw]';
    omega_ref = [omega_x omega_y omega_z]';
%     omega_dot_ref = [omega_dot_x omega_dot_y omega_dot_z]';
end

% Reference over the time window for NMPC
REF(:, i) = [ x y z ...     % p
              x_dot y_dot z_dot ...     % p_dot
              roll pitch yaw ...    % eta
              omega_x omega_y omega_z ...   % omega
              q1r   q2r  q3r...
              dq1r  dq2r dq3r ...
              x_ddot y_ddot z_ddot ...  % p_ddot
              domega_x domega_y domega_z ...  % omega_dot
              ddq1r  ddq2r ddq3r];
%               0*ones(nu_v,1)' ...   % alpha_dot
%               0*ones(nu_lambda,1)']'; %lambda_dot

end

%% Return output
ref = REF(:, 1:N);
% refN = REF(1:end-nu_v-nu_lambda, N+1);
refN = REF(1:nyN, N+1);

== matlab function MATMPC_SIMULINK_SPACEROBOT/NMPC Controller/Constraints subsystem/Constraints_Gen ==
  settings: sampleTime=sim_time_step
  data: lb output size=settings.size_b; settings parameter; indata parameter; states input size=settings.nx; ub output size=settings.size_b; lbu output size=settings.size_bu; ubu output size=settings.size_bu; lbx output size=settings.size_bx; ubx output size=settings.size_bx
function [lb, ub, lbu, ubu, lbx, ubx] = Constraints_Gen(settings, indata, states)


%% Importing 
% ... from  parameter `settings`
nu = settings.nu;
nu_lambda = settings.nu_lambda;
nu_v = settings.nu_v;
nbu = settings.nbu;
nbu_idx = settings.nbu_idx;
N = settings.N;

% ... from parameter `data`
%c_f = indata.model.c_f*ones(nu,1);
% omega_bar = indata.constraints.omega_bar;
% dot_omega_bar_max = indata.constraints.dot_omega_bar_max;
% dot_omega_bar_min = indata.constraints.dot_omega_bar_min;
% coeff_angular_acc = indata.constraints.coeff_angular_acc;
% coeff_angular_dec = indata.constraints.coeff_angular_dec;
%
%dot_alpha_min = indata.constraints.dot_alpha_min;
%dot_alpha_max = indata.constraints.dot_alpha_max;

f_min = indata.constraints.f_min ;
f_max = indata.constraints.f_max ;

% ... from input `states`
% State-dependent constraints
% F = zeros(0,1);
% for k = 0:nu-1
%     F = [F;states(13+k)];
% end
% f1 = states(13);
% f2 = states(14);
% f3 = states(15);
% f4 = states(16);
% f5 = states(17);
% f6 = states(18);

%% Variables definition

% vector F
% F = [f1; f2; f3; f4; f5; f6];

% Define the bounds of Delta U from equation:
%   dot_f(t) = 2 * kf * omega_i(t) * dot_omega_i(t),
%   where i is the i-th propeller 

%% Upper and lower bounds for general constraints 
% Dimensions of lb_g and ub_g should be equal to nc.
lb_g = [];
ub_g = [];

% Dimensions of lb_gN and ub_gN should be equal to ncN.
lb_gN = [];
ub_gN = [];

lb_g_rep = repmat(lb_g, N, 1);
ub_g_rep = repmat(ub_g, N, 1);

lb_temp = [lb_g_rep; lb_gN];
ub_temp = [ub_g_rep; ub_gN];

if isempty(lb_temp | ub_temp)
    
    lb = 0;
    ub = 0;

else
    
    lb = lb_temp;
    ub = ub_temp;
    
end

%% Lower and upper bounds for input 
% Dimensions of lb_u and ub_u should be equal to nbu.
lb_u = zeros(nbu, 1);
ub_u = zeros(nbu, 1);

lb_u(1:6) = f_min ;
ub_u(1:6) = f_max ;

%bounds for torques

lb_u(7:end) = -240;
ub_u(7:end) =  240;

% Propeller upper and lower bounds computation
% The bounds depend on current state of TiltHex. 
% This computation is repeated for each propellers
% dot_omega_temp_acc = zeros(nu_lambda, 1);
% dot_omega_temp_dec = zeros(nu_lambda, 1);
% 
% for i = 1:nu_lambda
% % At each value inside omega_bar corresponds an upper and lower bound of dot_omega_bar,
% % taken rispectively inside dot_omega_bar_max and dot_omega_bar_min.
% % First it is mandatory to understand in which interval is the force provided
% % by the i-th propeller; omega_bar values are translated into force
% % quantities by F = k_f*omega^2 relationship, then i-th propeller's force is 
% % compared to those value in order to understand in which interval the i-th 
% % propeller is working. Then, once found the interval, linear interpolation 
% % is used to adjust upper and lower bounds of extremity points of that
% % interval to the actual in-between point.
%         
%         % If less force is requested w.r.t. the first upper and lower
%         % bounds, then use first elements of omega_bar_min and _max
%         % AND ALSO (update Davide & Youssef 01/06/2021) set the lower and
%         % upper limits for the input equal to the same limits of the first
%         % (smaller) spinning velocity setpoint. 
%         % This is done to avoid the if a propeller is spinnijg with zero
%         % velocity also his bounds of acceleration are set to zero; we
%         % don't want this. Therefore, a minimum acceleration/deceleration
%         % is always guaranteed.
%         f_first_setpoint = c_f(i) * omega_bar(1)^2;
%         if (abs(F(i)) <= f_first_setpoint)
%             dot_omega_temp_acc(i) = dot_omega_bar_max(1);
%             dot_omega_temp_dec(i) = dot_omega_bar_min(1);
%             ub_u(i) = 2 * sqrt(f_first_setpoint * c_f(i)) * dot_omega_bar_max(1);
%             lb_u(i) = 2 * sqrt(f_first_setpoint * c_f(i)) * dot_omega_bar_min(1);
%         
%         % Otherwise you need to interpolate, depending at which omega the
%         % i-th propeller is spinning. 
%         elseif (abs(F(i)) > c_f(i) * omega_bar(1)^2 && abs(F(i)) <= c_f(i) * omega_bar(2)^2)
%             dot_omega_temp_acc(i) = (coeff_angular_acc(1) * (sqrt(abs(F(i)) / c_f(i)) - omega_bar(2)) + dot_omega_bar_max(2));
%             dot_omega_temp_dec(i) = (coeff_angular_dec(1) * (sqrt(abs(F(i)) / c_f(i)) - omega_bar(2)) + dot_omega_bar_min(2));
%             ub_u(i)= 2 * sqrt(abs(F(i)) * c_f(i)) * dot_omega_temp_acc(i);
%             lb_u(i)= 2 * sqrt(abs(F(i)) * c_f(i)) * dot_omega_temp_dec(i);
%             
%         elseif (abs(F(i)) > c_f(i) * omega_bar(2)^2 && abs(F(i)) <= c_f(i) * omega_bar(3)^2)
%             dot_omega_temp_acc(i) = (coeff_angular_acc(2) * (sqrt(abs(F(i)) / c_f(i)) - omega_bar(3)) + dot_omega_bar_max(3));
%             dot_omega_temp_dec(i) = (coeff_angular_dec(2) * (sqrt(abs(F(i)) / c_f(i)) - omega_bar(3)) + dot_omega_bar_min(3));
%             ub_u(i) = 2 * sqrt(abs(F(i)) * c_f(i)) * dot_omega_temp_acc(i);
%             lb_u(i) = 2 * sqrt(abs(F(i)) * c_f(i)) * dot_omega_temp_dec(i);
%         
%         elseif (abs(F(i)) > c_f(i) * omega_bar(3)^2 && abs(F(i)) <= c_f(i) * omega_bar(4)^2)
%             dot_omega_temp_acc(i) = (coeff_angular_acc(3) * (sqrt(abs(F(i)) / c_f(i)) - omega_bar(4)) + dot_omega_bar_max(4));
%             dot_omega_temp_dec(i) = (coeff_angular_dec(3) * (sqrt(abs(F(i)) / c_f(i)) - omega_bar(4)) + dot_omega_bar_min(4));
%             ub_u(i) = 2 * sqrt(abs(F(i)) * c_f(i)) * dot_omega_temp_acc(i);
%             lb_u(i) = 2 * sqrt(abs(F(i)) * c_f(i)) * dot_omega_temp_dec(i);
%         
%         elseif (abs(F(i)) > c_f(i) * omega_bar(4)^2 && abs(F(i)) <= c_f(i) * omega_bar(5)^2)
%             dot_omega_temp_acc(i) = (coeff_angular_acc(4) * (sqrt(abs(F(i)) / c_f(i)) - omega_bar(5)) + dot_omega_bar_max(5));
%             dot_omega_temp_dec(i) = (coeff_angular_dec(4) * (sqrt(abs(F(i)) / c_f(i)) - omega_bar(5)) + dot_omega_bar_min(5));
%             ub_u(i)= 2 * sqrt(abs(F(i)) * c_f(i)) * dot_omega_temp_acc(i);
%             lb_u(i)= 2 * sqrt(abs(F(i)) * c_f(i)) * dot_omega_temp_dec(i);
%         
%         elseif (abs(F(i)) > c_f(i) * omega_bar(5)^2 && abs(F(i)) <= c_f(i) * omega_bar(6)^2)
%             dot_omega_temp_acc(i) = (coeff_angular_acc(5) * (sqrt(abs(F(i)) / c_f(i)) - omega_bar(6)) + dot_omega_bar_max(6));
%             dot_omega_temp_dec(i) = (coeff_angular_dec(5) * (sqrt(abs(F(i)) / c_f(i)) - omega_bar(6)) + dot_omega_bar_min(6));
%             ub_u(i) = 2 * sqrt(abs(F(i)) * c_f(i)) * dot_omega_temp_acc(i);
%             lb_u(i) = 2 * sqrt(abs(F(i)) * c_f(i)) * dot_omega_temp_dec(i);
%         
%         elseif (abs(F(i)) > c_f(i) * omega_bar(6)^2)
%             dot_omega_temp_acc(i) = (coeff_angular_acc(6) * (sqrt(abs(F(i)) / c_f(i)) - omega_bar(7)) + dot_omega_bar_max(7));
%             dot_omega_temp_dec(i) = (coeff_angular_dec(6) * (sqrt(abs(F(i)) / c_f(i)) - omega_bar(7)) + dot_omega_bar_min(7));
%             ub_u(i) = 2 * sqrt(abs(F(i)) * c_f(i)) * dot_omega_temp_acc(i);
%             lb_u(i) = 2 * sqrt(abs(F(i)) * c_f(i)) * dot_omega_temp_dec(i);
%         end
% end

%
% for i = nu_lambda+1:nu_lambda+nu_v
%     ub_u(i) = dot_alpha_max;
%     lb_u(i) = dot_alpha_min;   
% end
%

lbu_temp = -inf(nu, 1);
ubu_temp = inf(nu, 1);

for i = 1:nbu
    lbu_temp(nbu_idx(i)) = lb_u(i);
    ubu_temp(nbu_idx(i)) = ub_u(i);
end

lbu = repmat(lbu_temp, 1, N);
ubu = repmat(ubu_temp, 1, N);

%% Lower and upper bounds for state 
lb_x = indata.constraints.lbx;
ub_x = indata.constraints.ubx;

if isempty(lb_x | ub_x)    
    lbx = zeros(1, N);
    ubx = zeros(1, N);
else
    lbx = repmat(lb_x, 1, N);
    ubx = repmat(ub_x, 1, N);
end

% disp('states')
% disp(states)
% disp('lowbound states')
% disp(lb_x)

end
